simulink model "OL_Adaptive_Integral_Control_TEST"  (R2021b)
settings: Solver=ode4  StartTime=0.0  StopTime=60  FixedStep=1e-3  RelTol=1e-3
settings Model: Creator=hellb  LastModifiedBy=hellb

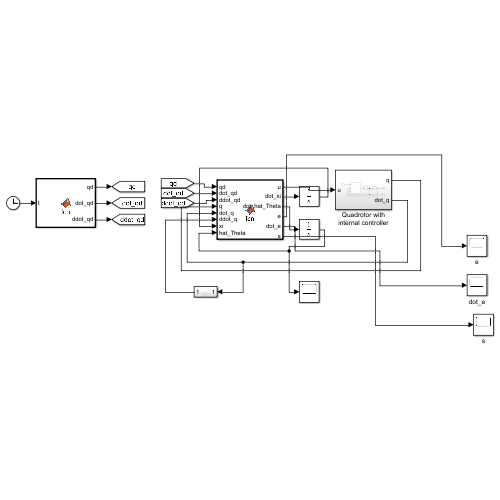
[thumbnail: Simulink's stored preview of the top-level diagram]
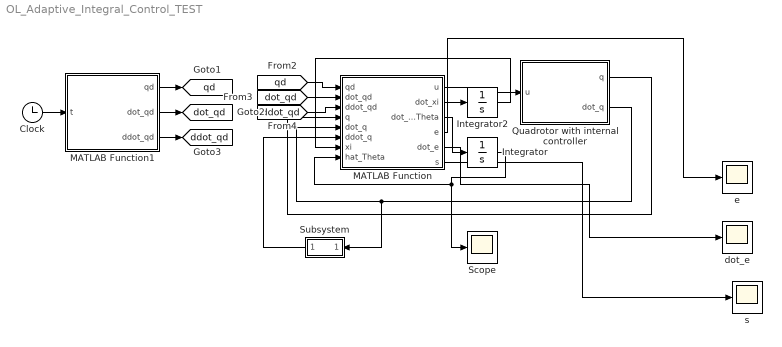
== system OL_Adaptive_Integral_Control_TEST ==
  Clock : Clock
  Integrator : Integrator  InitialCondition=0.65*[0.0632; 0.0632; 0.0943; 0.4202; 0.0013; 0.0013; 0.1334; 0.5898]
  Integrator2 : Integrator  InitialCondition=[0;0;0;0]
  MATLAB Function : MATLAB Function  TreatAsAtomicUnit=on
  MATLAB Function1 : MATLAB Function  TreatAsAtomicUnit=on
  Quadrotor with internal controller : Subsystem
  Scope : Scope
  Subsystem : Subsystem
  dot_e : Scope
  e : Scope
  s : Scope
  tag scope: ddot_qd=global, dot_qd=global, qd=global
  wires:
  MATLAB Function/5(dot_e) -> dot_e/1
  [qd] -> MATLAB Function/1(qd)
  MATLAB Function/2(dot_xi) -> Integrator2/1
  MATLAB Function1/3(ddot_qd) -> [ddot_qd]
  [dot_qd] -> MATLAB Function/2(dot_qd)
  Integrator2/1 -> MATLAB Function/7(xi)
  [ddot_qd] -> MATLAB Function/3(ddot_qd)
  MATLAB Function1/2(dot_qd) -> [dot_qd]
  MATLAB Function1/1(qd) -> [qd]
  Clock/1 -> MATLAB Function1/1(t)
  MATLAB Function/3(dot_hat_Theta) -> Integrator/1
  Quadrotor with internal controller/1(q) -> MATLAB Function/4(q)
  Integrator/1 -> Scope/1, MATLAB Function/8(hat_Theta)
  MATLAB Function/1(u) -> Quadrotor with internal controller/1(u)
  Quadrotor with internal controller/2(dot_q) -> MATLAB Function/5(dot_q), Subsystem/1(In1)
  MATLAB Function/4(e) -> e/1
  MATLAB Function/6(s) -> s/1
  Subsystem/1(Out1) -> MATLAB Function/6(ddot_q)

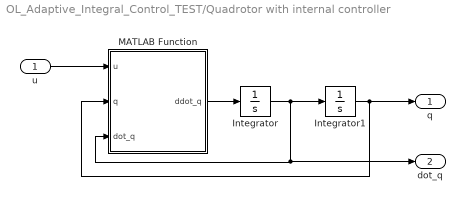
== system OL_Adaptive_Integral_Control_TEST/Quadrotor with internal controller ==
  u : Inport
  Integrator : Integrator  InitialCondition=[0;0;0;0]
  Integrator1 : Integrator  InitialCondition=[0;0;0.3;0]
  MATLAB Function : MATLAB Function  TreatAsAtomicUnit=on
  q : Outport  VectorParamsAs1DForOutWhenUnconnected=off
  dot_q : Outport  Port=2  VectorParamsAs1DForOutWhenUnconnected=off
  wires:
  Integrator/1 -> dot_q/1, MATLAB Function/3(dot_q), Integrator1/1
  Integrator1/1 -> q/1, MATLAB Function/2(q)
  MATLAB Function/1(ddot_q) -> Integrator/1
  u/1 -> MATLAB Function/1(u)

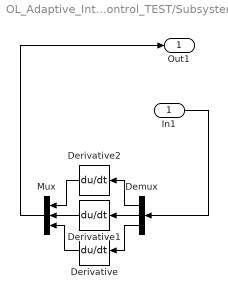
== system OL_Adaptive_Integral_Control_TEST/Subsystem ==
  In1 : Inport
  Demux : Demux  Outputs=3
  Derivative : Derivative
  Derivative1 : Derivative
  Derivative2 : Derivative
  Mux : Mux  Inputs=3
  Out1 : Outport
  wires:
  In1/1 -> Demux/1
  Derivative/1 -> Mux/3
  Derivative1/1 -> Mux/2
  Demux/2 -> Derivative1/1
  Demux/1 -> Derivative2/1
  Demux/3 -> Derivative/1
  Derivative2/1 -> Mux/1
  Mux/1 -> Out1/1

== matlab function OL_Adaptive_Integral_Control_TEST/MATLAB Function ==
  data: qd input; u output; dot_xi output; dot_qd input; ddot_qd input; q input; dot_q input; ddot_q input; xi input; dot_hat_Theta output; e output; hat_Theta input; dot_e output; s output
function [u, dot_xi, dot_hat_Theta, e, dot_e, s] = fcn(qd, dot_qd, ddot_qd, q, dot_q, ddot_q, xi, hat_Theta)

K_P = diag([1.5 1.5 2.5 2]);
% Ks = 0.25*K_P;
Kd = 0*K_P;
Ki = 1*diag([0.001 0.001 0.005 0.006]);

% Gamma = Ks\(K_P - Ki);
Gamma = diag([2.5 2.5 4 3]);
Ks = 3*Gamma;

N  = 50*1.8*diag(ones(8,1));
k  = 1*0.09;

psi   = q(4);
e     = qd - q;
dot_e = dot_qd - dot_q;
ddot_e = ddot_qd - ddot_q;
s     = Gamma*e + dot_e;
dot_s = Gamma*dot_e + ddot_e;
f1    = Gamma*dot_e + ddot_qd;
f2    = dot_qd - dot_e;

T  = [cos(psi)  sin(psi) 0 0
      sin(psi) -cos(psi) 0 0
      0         0        1 0
      0         0        0 1];

Phi = [f1(1) 0 0 0 f2(1) 0 0 0
       0 f1(2) 0 0 0 f2(2) 0 0
       0 0 f1(3) 0 0 0 f2(3) 0
       0 0 0 f1(4) 0 0 0 f2(4)];

u      = T\(Ks*s + Ki*xi + Kd*dot_s + Phi*hat_Theta);
dot_xi = s;
dot_hat_Theta = N*(Phi'*s - k*norm(s)*hat_Theta);

== matlab function OL_Adaptive_Integral_Control_TEST/Quadrotor with internal controller/MATLAB Function ==
  data: u input; ddot_q output; q input; dot_q input
function ddot_q = fcn(u, q, dot_q)
psi = q(4);
% Parametros tomados del articulo de Adaptive GRNNC
% correspondientes al QBall 2 de Quanser.
g = 9.81;
m = 1.79;
tht_max = deg2rad(92.35);
phi_max = deg2rad(92.35);
dotz_max = 7.7168;
dotpsi_max = deg2rad(99.2730);
tau_dotz   = 0.728;
tau_dotpsi = 0.728;
dx = 0.02;
dy = 0.02;
dz = 0.04;
dpsi = 0.03;
% %%%%%%%%%%%%%%%%%%%%%%%%%%%%%%%%%%%%%%%%%%%%%%%%%
Ku = diag([g*tht_max g*phi_max dotz_max/tau_dotz dotpsi_max/tau_dotpsi]);
Kv = diag([dx dy ((1/tau_dotz)+dz) ((1/tau_dotpsi)+dpsi)]);

T  = [cos(psi)  sin(psi) 0 0
      sin(psi) -cos(psi) 0 0
      0         0        1 0
      0         0        0 1];
  
ddot_q = T*Ku*u - Kv*dot_q;

== matlab function OL_Adaptive_Integral_Control_TEST/MATLAB Function1 ==
  data: t input; qd output; dot_qd output; ddot_qd output

function [qd, dot_qd, ddot_qd] = fcn(t)

xfreq = 2*pi/4;
yfreq = 2*pi/8;
zfreq = 2*pi/8;
psifreq = 2*pi/8;
xamp = 0.5;
yamp = 1;
zamp = 0.1;
psiamp = deg2rad(30);
h = 1;
hf = h - zamp + 0.002477;
h0 = 0.3;
b = 0.05;

if t <= 2*pi
qd = [xamp*sin(xfreq*t)*(1-exp(-0.1*t^3))
      yamp*cos(yfreq*t)*(1-exp(-0.1*t^3))
      hf - exp(-b*t^3)*(hf - h0)
      psiamp*sin(psifreq*t)*(1-exp(-0.1*t^3))];

dot_qd = [3*b*t^2*xamp*exp(-b*t^3)*sin(t*xfreq) - xamp*xfreq*cos(t*xfreq)*(exp(-b*t^3) - 1)
          yamp*yfreq*sin(t*yfreq)*(exp(-b*t^3) - 1) + 3*b*t^2*yamp*exp(-b*t^3)*cos(t*yfreq)
          3*b*t^2*exp(-b*t^3)*(hf - h0)
          3*b*t^2*psiamp*exp(-b*t^3)*sin(t*psifreq) - psiamp*psifreq*cos(t*psifreq)*(exp(-b*t^3) - 1)];
ddot_qd = [xamp*xfreq^2*sin(t*xfreq)*(exp(-b*t^3) - 1) - 9*b^2*t^4*xamp*exp(-b*t^3)*sin(t*xfreq) + 6*b*t*xamp*exp(-b*t^3)*sin(t*xfreq) + 6*b*t^2*xamp*xfreq*exp(-b*t^3)*cos(t*xfreq)
           yamp*yfreq^2*cos(t*yfreq)*(exp(-b*t^3) - 1) - 9*b^2*t^4*yamp*exp(-b*t^3)*cos(t*yfreq) + 6*b*t*yamp*exp(-b*t^3)*cos(t*yfreq) - 6*b*t^2*yamp*yfreq*exp(-b*t^3)*sin(t*yfreq)
           6*b*t*exp(-b*t^3)*(hf - h0) - 9*b^2*t^4*exp(-b*t^3)*(hf - h0)
           psiamp*psifreq^2*sin(t*psifreq)*(exp(-b*t^3) - 1) - 9*b^2*t^4*psiamp*exp(-b*t^3)*sin(t*psifreq) + 6*b*t*psiamp*exp(-b*t^3)*sin(t*psifreq) + 6*b*t^2*psiamp*psifreq*exp(-b*t^3)*cos(t*psifreq)];
else
qd = [xamp*sin(xfreq*t)
      yamp*cos(yfreq*t)
      h + zamp*sin(zfreq*t)
      psiamp*sin(psifreq*t)];

dot_qd = [xfreq*xamp*cos(xfreq*t)
          -yfreq*yamp*sin(yfreq*t)
          zamp*zfreq*cos(t*zfreq)
          psifreq*psiamp*cos(psifreq*t)];
ddot_qd = [-xfreq^2*xamp*sin(xfreq*t)
           -yfreq^2*yamp*cos(yfreq*t)
           -zamp*zfreq^2*sin(t*zfreq)
           -psifreq^2*psiamp*sin(psifreq*t)];
end
